simulink model "RoadRunnerSceneImport"  (R2022b)
settings: Solver=VariableStepAuto  StartTime=0.0  StopTime=10  RelTol=1e-3
libraries: visionsinks x3, sim3dautolib x2, sim3dcameralib x1, sim3dlib x1, drivingsim3d x1
settings Model: Creator=The MathWorks, Inc.  LastModifiedBy=Administrator

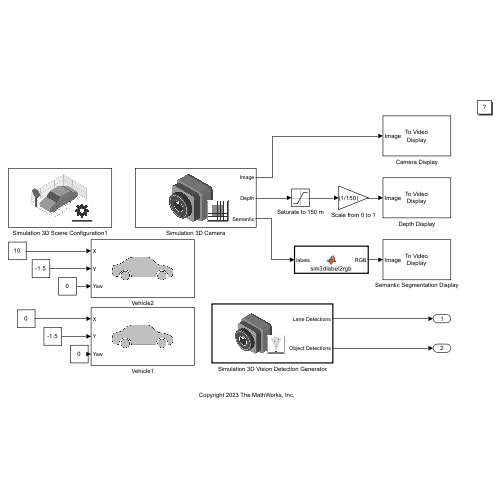
[thumbnail: Simulink's stored preview of the top-level diagram]
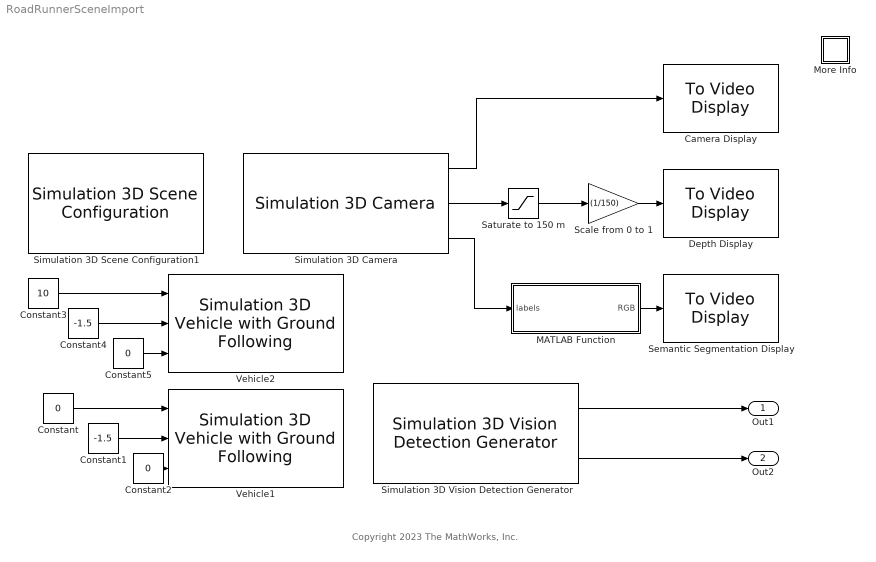
== system RoadRunnerSceneImport ==
  note: Copyright 2023 The MathWorks, Inc.
  Camera Display : visionsinks/To Video Display  windowSizeMode=Normal  openAtMdlStart=on  fullScreen=off  videoWindowX=536805376  videoWindowY=536805376  saveWindowSize=off  videoWindowWidth=1280  videoWindowHeight=720  inputColorFormat=RGB  inputType=Obsolete  imagePorts=One multidimensional signal  OutputDevice=On-screen video monitor  dataOrg=Column-major  isWindowOpen=off
  Constant : Constant  Value=0
  Constant1 : Constant  Value=-1.5
  Constant2 : Constant  Value=0
  Constant3 : Constant  Value=10
  Constant4 : Constant  Value=-1.5
  Constant5 : Constant  Value=0
  Depth Display : visionsinks/To Video Display  windowSizeMode=Normal  openAtMdlStart=on  fullScreen=off  videoWindowX=536805376  videoWindowY=536805376  saveWindowSize=off  videoWindowWidth=1280  videoWindowHeight=720  inputColorFormat=RGB  inputType=Obsolete  imagePorts=One multidimensional signal  OutputDevice=On-screen video monitor  dataOrg=Column-major  isWindowOpen=off
  MATLAB Function : MATLAB Function  TreatAsAtomicUnit=on
  More Info : Subsystem
      settings: OpenFcn=showExample('sim3d/ViewSemanticSegmentationAndVisionDetectionInRRSceneExample')
      mask Display: disp('?')
  Saturate to 150 m : Saturate  UpperLimit=150  LowerLimit=0
  Scale from 0 to 1 : Gain  Gain=(1/150)
  Semantic Segmentation Display : visionsinks/To Video Display  windowSizeMode=Normal  openAtMdlStart=on  fullScreen=off  videoWindowX=536805376  videoWindowY=536805376  saveWindowSize=off  videoWindowWidth=1280  videoWindowHeight=720  inputColorFormat=RGB  inputType=Obsolete  imagePorts=One multidimensional signal  OutputDevice=On-screen video monitor  dataOrg=Column-major  isWindowOpen=off
  Simulation 3D Camera : sim3dcameralib/Simulation 3D Camera  Priority=1  sensorTag=Sim3dSensor3  sensorId=3  sensorName=Sim3dSensor3  vehTagList={'Scene Origin';'SimulinkVehicle1';'SimulinkVehicle2'}  vehTag=SimulinkVehicle1  mountLoc=Origin  offsetFlag=on  tmountOffset=[-6, 0, 2]  extTmount=off  rmountOffset=[0, 10, 0]  extRmount=off  FocalLength=[1109, 1109]  OpticalCenter=[640, 360]  ImageSize=[720, 1280]  RadialDistortion=[0, 0]  TangentialDistortion=[0, 0]  SensorSkew=0  DepthOutportEnabled=on  SemanticOutportEnabled=on  TransformOutportEnabled=off  SampleTime=-1  mountPoint=[-6 0 2]  mountOrientation=[0 -10 0]  aMode=3  ID=3
      settings: LibrarySourceBlock=drivingsim3d/Simulation 3D Camera
  Simulation 3D Scene Configuration1 : sim3dlib/Simulation 3D Scene Configuration  Priority=0  ProjectFormat=RoadRunner  SceneDesc=Straight road  ProjectName=D:\software\matlab_2023b\toolbox\shared\sim3d_projects\automotive_project_windows\UE\WindowsNoEditor\VehicleSimulation.exe  ScenePath=/Game/Maps/HwStrght  RoadRunnerProjectPath=.\Data\sim3dRoad.fbx  EnableOpenDRIVE=off  vehTagList={'Scene Origin';'SimulinkVehicle1';'SimulinkVehicle2'}  vehTag=SimulinkVehicle1  FreeCameraInitialTranslation=[0, 0, 0]  FreeCameraDefaultInitialTranslation=[-6, 0, 2]  FreeCameraInitialRotation=[0, 0, 0]  FreeCameraDefaultInitialRotation=[0, -15, 0]  OpVisEn=off  Ts=1/60  EnableWindow=on  EnableRemoteAccess=off  EnableWeather=off  SunAltitude=40.0  SunAzimuth=90  clouds=10  wind=1  fog=0  rain=0  EnableGeospatial=off  OriginHeight=200  OriginLatitude=40.744652  OriginLongitude=-73.988864  MapStyle=Aerial  AdditionalAssetIDs=[]  UseAdvancedSunSky=off  SolarTime=11  TimeZone=-5  Day=21  Month=9  Year=2022  UseDaylightSavingTime=on  DSTStartDay=10  DSTStartMonth=3  DSTEndDay=3  DSTEndMonth=11  DSTSwitchHour=2  sensorTag=MainCamera2  sensorId=2  sensorName=MainCamera2  mountLoc=Origin  offsetFlag=off  tmountOffset=[0, 0, 0]  rmountOffset=[0, 0, 0]  HorizontalResolution=1280  VerticalResolution=720  HorizontalFOV=60  mountPoint=[0 0 0]  mountOrientation=[0 0 0]  aMode=3  ID=2  GeoTrigger=Inactive
      settings: LibrarySourceBlock=drivingsim3d/Simulation 3D Scene Configuration
  Simulation 3D Vision Detection Generator : drivingsim3d/Simulation 3D Vision Detection Generator  Priority=1  sensorTag=Sim3dSensor255  sensorId=4  sensorName=Sim3dSensor255  vehTagList={'Scene Origin';'SimulinkVehicle1';'SimulinkVehicle2'}  vehTag=SimulinkVehicle1  mountLoc=Rearview mirror  offsetFlag=off  tmountOffset=[0, 0, 1.5]  rmountOffset=[0, 15, 0]  DetectorOutput=Lanes and objects  MaxNumDetections=50  MaxNumLanes=30  laneSampleDistances=0:0.5:9.5  BusNameSource=Auto  BusName=BusObjectDetections  BusName2Source=Auto  BusName2=BusLaneDetections  MaxRange=150  BoundingBoxAccuracy=5  ProcessNoiseIntensity=5  MaxSpeed=50  MaxAllowedOcclusion=0.5  MinObjectImageSize=[ 15, 15 ]  DetectionProbability=0.9  FalsePositivesPerImage=0.1  MinLaneImageSize=[ 20, 3 ]  LaneBoundaryAccuracy=3  HasNoise=on  InitialSeedSource=Repeatable  InitialSeed=1  uniqueActorIdentifier=[]  actorClassInteger=0  cuboidLength=4.7  cuboidWidth=1.8  cuboidHeight=1.4  rotationalCenter={[-1.35, 0, 0]}  focalLength=[800, 800]  opticalCenter=[320, 240]  imageSize=[480, 640]  radialDistortionCoefficients=[0, 0]  tangentialDistortionCoefficients=[0, 0]  cameraAxisSkew=0  actorTruthOutportEnabled=off  laneTruthOutportEnabled=off  SampleTime=-1  checkedSampleTime=0.016667  mountPoint=[0.319999992847443 0 1.19000005722046]  mountOrientation=[0 0 0]  aMode=3  ID=4
  Vehicle1 : sim3dautolib/Simulation 3D Vehicle with Ground Following  Priority=-1  PassVehMesh=Muscle car  MeshPath=/MathWorksAutomotiveContent/Vehicles/Muscle/Meshes/SK_MuscleCar.SK_MuscleCar  TrackWidth=1.9  WheelBase=3  WheelRadius=0.35  VehColor=Red  InitialPos=[0, -1.5, 0]  InitialRot=[0, 0, 0]  ActorName=SimulinkVehicle1  SampleTime=-1  ActorType=SimulinkVehicle  ID=1  aMode=3  ActorTag=SimulinkVehicle1  CoordinateScheme=ISO  VehLightsControl=off  HeadlightColor=[ 1, 1, 1 ]  HighBeamIntensity=100000  LowBeamIntensity=60000  HighBeamConeAngle=70  LowBeamConeAngle=70  LeftHeadlightOrientation=[ 0, 0 ]  RightHeadlightOrientation=[ 0, 0 ]  BrakelightIntensity=500  ReverselightIntensity=500  SignallightIntensity=500  SignallightPeriod=1  SignalPulseWidth=50  TransformOutportEnabled=off
      settings: LibrarySourceBlock=drivingsim3d/Simulation 3D Vehicle with Ground Following
  Vehicle2 : sim3dautolib/Simulation 3D Vehicle with Ground Following  Priority=-1  PassVehMesh=Muscle car  MeshPath=/MathWorksAutomotiveContent/Vehicles/Muscle/Meshes/SK_MuscleCar.SK_MuscleCar  TrackWidth=1.9  WheelBase=3  WheelRadius=0.35  VehColor=Red  InitialPos=[10, -1.5, 0]  InitialRot=[0, 0, 0]  ActorName=SimulinkVehicle2  SampleTime=-1  ActorType=SimulinkVehicle  ID=2  aMode=3  ActorTag=SimulinkVehicle2  CoordinateScheme=ISO  VehLightsControl=off  HeadlightColor=[ 1, 1, 1 ]  HighBeamIntensity=100000  LowBeamIntensity=60000  HighBeamConeAngle=70  LowBeamConeAngle=70  LeftHeadlightOrientation=[ 0, 0 ]  RightHeadlightOrientation=[ 0, 0 ]  BrakelightIntensity=500  ReverselightIntensity=500  SignallightIntensity=500  SignallightPeriod=1  SignalPulseWidth=50  TransformOutportEnabled=off
      settings: LibrarySourceBlock=drivingsim3d/Simulation 3D Vehicle with Ground Following
  Out1 : Outport
  Out2 : Outport  Port=2
  wires:
  Simulation 3D Vision Detection Generator/1 -> Out1/1
  Simulation 3D Vision Detection Generator/2 -> Out2/1
  Constant/1 -> Vehicle1/1
  Constant1/1 -> Vehicle1/2
  Constant2/1 -> Vehicle1/3
  Constant3/1 -> Vehicle2/1
  Constant4/1 -> Vehicle2/2
  Constant5/1 -> Vehicle2/3
  Simulation 3D Camera/3 -> MATLAB Function/1(labels)
  Scale from 0 to 1/1 -> Depth Display/1
  MATLAB Function/1(RGB) -> Semantic Segmentation Display/1
  Simulation 3D Camera/2 -> Saturate to 150 m/1
  Simulation 3D Camera/1 -> Camera Display/1
  Saturate to 150 m/1 -> Scale from 0 to 1/1

== system RoadRunnerSceneImport/More Info ==

== matlab function RoadRunnerSceneImport/MATLAB Function ==
  data: labels input; RGB output
function RGB = sim3dlabel2rgb(labels)
% Convert semantic segmentation map captured during 3D simulation to RGB
% color image.

% Declare label2rgb function.
coder.extrinsic('label2rgb');

% Preallocate memory for RGB matrix.
RGB = coder.nullcopy(zeros(size(labels,1),size(labels,2),3,class(labels)));

% Define colormap using 3D simulation label IDs.
cmap = sim3dColormap;

% Convert labels to RGB color image.
RGB = label2rgb(labels, cmap);
